simulink model "ErskineMultiDroneFormation"  (R2020b)
settings: Solver=FixedStepAuto  StartTime=0.0  StopTime=Tsim  FixedStep=sim_dt  RelTol=1e-3
values from neighbouring files (symbols this model uses):
  controller_rate = 50    [MultiQuadInit.m]
  drone_params = setDefaultDroneParams(nDrones)    [MultiQuadInit.m]
  dt_p = 0.2    [MultiQuadInit.m]    (also in setSimConditions.m)
  edges = [1,2 ... (first row only)    [MultiQuadInit.m]    (also in setSimConditions.m)
  g = 9.81    [MultiQuadInit.m]
  N_p = 5    [MultiQuadInit.m]    (also in setSimConditions.m)
  nDrones = 3    [MultiQuadInit.m]
  omega0 = zeros(3,nDrones)    [MultiQuadInit.m]    (also in setSimConditions.m)
  p0 = scale*(rand(3,nDrones) - [0.5;0.5;0])    [MultiQuadInit.m]    (also in setSimConditions.m = scale*(rand(3,nDrones) - [1/2;1/2;0]))
  q0 = zeros(4,nDrones); q0(1,:) = ones(1,nDrones)    [MultiQuadInit.m]    (also in setSimConditions.m)
  sim_dt = 0.005    [MultiQuadInit.m]
  v0 = zeros(3, nDrones)    [MultiQuadInit.m]    (also in setSimConditions.m)
undefined symbols (not defined in the file or in its folder): camera_noise
libraries: vrlib x13
(part 2 of 4)

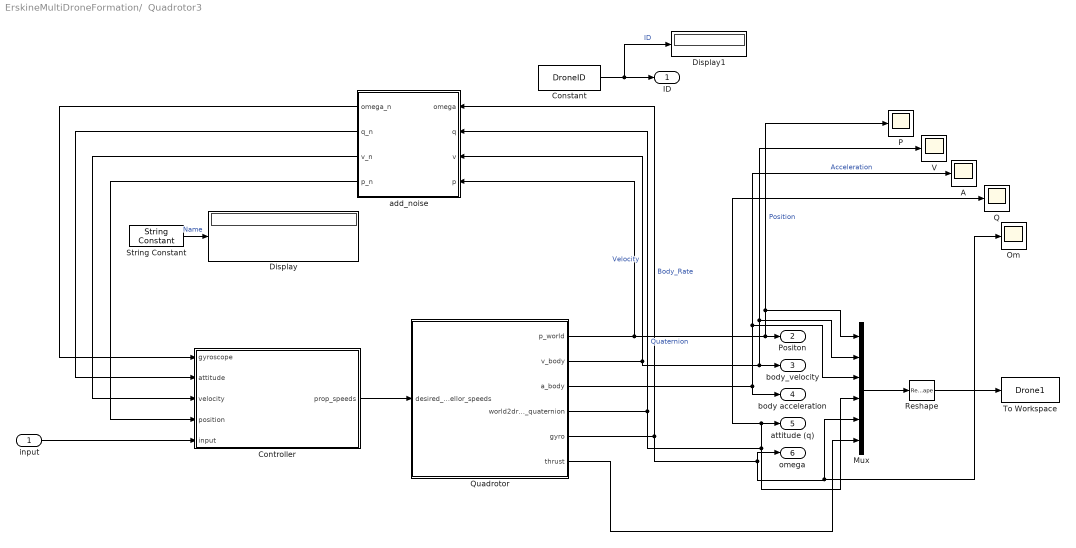
== system ErskineMultiDroneFormation/  Quadrotor3 ==
  input : Inport
  A : Scope
  Constant : Constant  Value=DroneID
  Controller : Subsystem
      mask Display: image('Format/flightController.png'); % Use "Edit Image" on toolstrip to change.
  Display : Display
  Display1 : Display
  Mux : Mux  Inputs=6
  Om : Scope
  P : Scope
  Q : Scope
  Quadrotor : Subsystem
      mask Display: image('droneHardware.jpeg'); % Use "Edit Image" on toolstrip to change.
  Reshape : Reshape
  String Constant : StringConstant  String=DroneName
  To Workspace : ToWorkspace  VariableName=Drone1  SaveFormat=Timeseries  SampleTime=-1
  V : Scope
  add_noise : MATLAB Function  TreatAsAtomicUnit=on
  ID : Outport
  Positon : Outport  Port=2
  body_velocity : Outport  Port=3
  body acceleration : Outport  Port=4
  attitude (q) : Outport  Port=5
  omega : Outport  Port=6
  wires:
  Quadrotor/5(gyro) -> Om/1, Mux/5, omega/1, add_noise/1(omega)  "Body_Rate"
  Quadrotor/1(p_world) -> add_noise/4(p), P/1, Mux/1, Positon/1  "Position"
  Quadrotor/3(a_body) -> body acceleration/1, A/1, Mux/3  "Acceleration"
  Quadrotor/4(world2drone_quaternion) -> Q/1, attitude (q)/1, Mux/4, add_noise/2(q)  "Quaternion"
  Mux/1 -> Reshape/1
  Quadrotor/2(v_body) -> V/1, Mux/2, body_velocity/1, add_noise/3(v)  "Velocity"
  Quadrotor/6(thrust) -> Mux/6
  String Constant/1 -> Display/1  "Name"
  Constant/1 -> Display1/1, ID/1  "ID"
  Reshape/1 -> To Workspace/1
  add_noise/1(omega_n) -> Controller/1(gyroscope)
  add_noise/2(q_n) -> Controller/2(attitude)
  add_noise/3(v_n) -> Controller/3(velocity)
  add_noise/4(p_n) -> Controller/4(position)
  input/1 -> Controller/5(input)
  Controller/1(prop_speeds) -> Quadrotor/1(desired_propellor_speeds)

== system ErskineMultiDroneFormation/  Quadrotor4 ==
  input : Inport
  A : Scope
  Constant : Constant  Value=DroneID
  Controller : Subsystem
      mask Display: image('Format/flightController.png'); % Use "Edit Image" on toolstrip to change.
  Display : Display
  Display1 : Display
  Mux : Mux  Inputs=6
  Om : Scope
  P : Scope
  Q : Scope
  Quadrotor : Subsystem
      mask Display: image('droneHardware.jpeg'); % Use "Edit Image" on toolstrip to change.
  Reshape : Reshape
  String Constant : StringConstant  String=DroneName
  To Workspace : ToWorkspace  VariableName=Drone5  SaveFormat=Timeseries  SampleTime=-1
  V : Scope
  add_noise : MATLAB Function  TreatAsAtomicUnit=on
  ID : Outport
  Positon : Outport  Port=2
  body_velocity : Outport  Port=3
  body acceleration : Outport  Port=4
  attitude (q) : Outport  Port=5
  omega : Outport  Port=6
  wires:
  Quadrotor/5(gyro) -> Om/1, Mux/5, omega/1, add_noise/1(omega)  "Body_Rate"
  Quadrotor/1(p_world) -> add_noise/4(p), P/1, Mux/1, Positon/1  "Position"
  Quadrotor/3(a_body) -> body acceleration/1, A/1, Mux/3  "Acceleration"
  Quadrotor/4(world2drone_quaternion) -> Q/1, attitude (q)/1, Mux/4, add_noise/2(q)  "Quaternion"
  Mux/1 -> Reshape/1
  Quadrotor/2(v_body) -> V/1, Mux/2, body_velocity/1, add_noise/3(v)  "Velocity"
  Quadrotor/6(thrust) -> Mux/6
  String Constant/1 -> Display/1  "Name"
  Constant/1 -> Display1/1, ID/1  "ID"
  Reshape/1 -> To Workspace/1
  add_noise/1(omega_n) -> Controller/1(gyroscope)
  add_noise/2(q_n) -> Controller/2(attitude)
  add_noise/3(v_n) -> Controller/3(velocity)
  add_noise/4(p_n) -> Controller/4(position)
  input/1 -> Controller/5(input)
  Controller/1(prop_speeds) -> Quadrotor/1(desired_propellor_speeds)

== system ErskineMultiDroneFormation/  Quadrotor5 ==
  input : Inport
  A : Scope
  Constant : Constant  Value=DroneID
  Controller : Subsystem
      mask Display: image('Format/flightController.png'); % Use "Edit Image" on toolstrip to change.
  Display : Display
  Display1 : Display
  Mux : Mux  Inputs=6
  Om : Scope
  P : Scope
  Q : Scope
  Quadrotor : Subsystem
      mask Display: image('droneHardware.jpeg'); % Use "Edit Image" on toolstrip to change.
  Reshape : Reshape
  String Constant : StringConstant  String=DroneName
  To Workspace : ToWorkspace  VariableName=Drone6  SaveFormat=Timeseries  SampleTime=-1
  V : Scope
  add_noise : MATLAB Function  TreatAsAtomicUnit=on
  ID : Outport
  Positon : Outport  Port=2
  body_velocity : Outport  Port=3
  body acceleration : Outport  Port=4
  attitude (q) : Outport  Port=5
  omega : Outport  Port=6
  wires:
  Quadrotor/5(gyro) -> Om/1, Mux/5, omega/1, add_noise/1(omega)  "Body_Rate"
  Quadrotor/1(p_world) -> add_noise/4(p), P/1, Mux/1, Positon/1  "Position"
  Quadrotor/3(a_body) -> body acceleration/1, A/1, Mux/3  "Acceleration"
  Quadrotor/4(world2drone_quaternion) -> Q/1, attitude (q)/1, Mux/4, add_noise/2(q)  "Quaternion"
  Mux/1 -> Reshape/1
  Quadrotor/2(v_body) -> V/1, Mux/2, body_velocity/1, add_noise/3(v)  "Velocity"
  Quadrotor/6(thrust) -> Mux/6
  String Constant/1 -> Display/1  "Name"
  Constant/1 -> Display1/1, ID/1  "ID"
  Reshape/1 -> To Workspace/1
  add_noise/1(omega_n) -> Controller/1(gyroscope)
  add_noise/2(q_n) -> Controller/2(attitude)
  add_noise/3(v_n) -> Controller/3(velocity)
  add_noise/4(p_n) -> Controller/4(position)
  input/1 -> Controller/5(input)
  Controller/1(prop_speeds) -> Quadrotor/1(desired_propellor_speeds)

== system ErskineMultiDroneFormation/  Quadrotor6 ==
  input : Inport
  A : Scope
  Constant : Constant  Value=DroneID
  Controller : Subsystem
      mask Display: image('Format/flightController.png'); % Use "Edit Image" on toolstrip to change.
  Display : Display
  Display1 : Display
  Mux : Mux  Inputs=6
  Om : Scope
  P : Scope
  Q : Scope
  Quadrotor : Subsystem
      mask Display: image('droneHardware.jpeg'); % Use "Edit Image" on toolstrip to change.
  Reshape : Reshape
  String Constant : StringConstant  String=DroneName
  To Workspace : ToWorkspace  VariableName=Drone4  SaveFormat=Timeseries  SampleTime=-1
  V : Scope
  add_noise : MATLAB Function  TreatAsAtomicUnit=on
  ID : Outport
  Positon : Outport  Port=2
  body_velocity : Outport  Port=3
  body acceleration : Outport  Port=4
  attitude (q) : Outport  Port=5
  omega : Outport  Port=6
  wires:
  Quadrotor/5(gyro) -> Om/1, Mux/5, omega/1, add_noise/1(omega)  "Body_Rate"
  Quadrotor/1(p_world) -> add_noise/4(p), P/1, Mux/1, Positon/1  "Position"
  Quadrotor/3(a_body) -> body acceleration/1, A/1, Mux/3  "Acceleration"
  Quadrotor/4(world2drone_quaternion) -> Q/1, attitude (q)/1, Mux/4, add_noise/2(q)  "Quaternion"
  Mux/1 -> Reshape/1
  Quadrotor/2(v_body) -> V/1, Mux/2, body_velocity/1, add_noise/3(v)  "Velocity"
  Quadrotor/6(thrust) -> Mux/6
  String Constant/1 -> Display/1  "Name"
  Constant/1 -> Display1/1, ID/1  "ID"
  Reshape/1 -> To Workspace/1
  add_noise/1(omega_n) -> Controller/1(gyroscope)
  add_noise/2(q_n) -> Controller/2(attitude)
  add_noise/3(v_n) -> Controller/3(velocity)
  add_noise/4(p_n) -> Controller/4(position)
  input/1 -> Controller/5(input)
  Controller/1(prop_speeds) -> Quadrotor/1(desired_propellor_speeds)

== system ErskineMultiDroneFormation/  Quadrotor7 ==
  input : Inport
  A : Scope
  Constant : Constant  Value=DroneID
  Controller : Subsystem
      mask Display: image('Format/flightController.png'); % Use "Edit Image" on toolstrip to change.
  Display : Display
  Display1 : Display
  Mux : Mux  Inputs=6
  Om : Scope
  P : Scope
  Q : Scope
  Quadrotor : Subsystem
      mask Display: image('droneHardware.jpeg'); % Use "Edit Image" on toolstrip to change.
  Reshape : Reshape
  String Constant : StringConstant  String=DroneName
  To Workspace : ToWorkspace  VariableName=Drone8  SaveFormat=Timeseries  SampleTime=-1
  V : Scope
  add_noise : MATLAB Function  TreatAsAtomicUnit=on
  ID : Outport
  Positon : Outport  Port=2
  body_velocity : Outport  Port=3
  body acceleration : Outport  Port=4
  attitude (q) : Outport  Port=5
  omega : Outport  Port=6
  wires:
  Quadrotor/5(gyro) -> Om/1, Mux/5, omega/1, add_noise/1(omega)  "Body_Rate"
  Quadrotor/1(p_world) -> add_noise/4(p), P/1, Mux/1, Positon/1  "Position"
  Quadrotor/3(a_body) -> body acceleration/1, A/1, Mux/3  "Acceleration"
  Quadrotor/4(world2drone_quaternion) -> Q/1, attitude (q)/1, Mux/4, add_noise/2(q)  "Quaternion"
  Mux/1 -> Reshape/1
  Quadrotor/2(v_body) -> V/1, Mux/2, body_velocity/1, add_noise/3(v)  "Velocity"
  Quadrotor/6(thrust) -> Mux/6
  String Constant/1 -> Display/1  "Name"
  Constant/1 -> Display1/1, ID/1  "ID"
  Reshape/1 -> To Workspace/1
  add_noise/1(omega_n) -> Controller/1(gyroscope)
  add_noise/2(q_n) -> Controller/2(attitude)
  add_noise/3(v_n) -> Controller/3(velocity)
  add_noise/4(p_n) -> Controller/4(position)
  input/1 -> Controller/5(input)
  Controller/1(prop_speeds) -> Quadrotor/1(desired_propellor_speeds)

== system ErskineMultiDroneFormation/  Quadrotor8 ==
  input : Inport
  A : Scope
  Constant : Constant  Value=DroneID
  Controller : Subsystem
      mask Display: image('Format/flightController.png'); % Use "Edit Image" on toolstrip to change.
  Display : Display
  Display1 : Display
  Mux : Mux  Inputs=6
  Om : Scope
  P : Scope
  Q : Scope
  Quadrotor : Subsystem
      mask Display: image('droneHardware.jpeg'); % Use "Edit Image" on toolstrip to change.
  Reshape : Reshape
  String Constant : StringConstant  String=DroneName
  To Workspace : ToWorkspace  VariableName=Drone9  SaveFormat=Timeseries  SampleTime=-1
  V : Scope
  add_noise : MATLAB Function  TreatAsAtomicUnit=on
  ID : Outport
  Positon : Outport  Port=2
  body_velocity : Outport  Port=3
  body acceleration : Outport  Port=4
  attitude (q) : Outport  Port=5
  omega : Outport  Port=6
  wires:
  Quadrotor/5(gyro) -> Om/1, Mux/5, omega/1, add_noise/1(omega)  "Body_Rate"
  Quadrotor/1(p_world) -> add_noise/4(p), P/1, Mux/1, Positon/1  "Position"
  Quadrotor/3(a_body) -> body acceleration/1, A/1, Mux/3  "Acceleration"
  Quadrotor/4(world2drone_quaternion) -> Q/1, attitude (q)/1, Mux/4, add_noise/2(q)  "Quaternion"
  Mux/1 -> Reshape/1
  Quadrotor/2(v_body) -> V/1, Mux/2, body_velocity/1, add_noise/3(v)  "Velocity"
  Quadrotor/6(thrust) -> Mux/6
  String Constant/1 -> Display/1  "Name"
  Constant/1 -> Display1/1, ID/1  "ID"
  Reshape/1 -> To Workspace/1
  add_noise/1(omega_n) -> Controller/1(gyroscope)
  add_noise/2(q_n) -> Controller/2(attitude)
  add_noise/3(v_n) -> Controller/3(velocity)
  add_noise/4(p_n) -> Controller/4(position)
  input/1 -> Controller/5(input)
  Controller/1(prop_speeds) -> Quadrotor/1(desired_propellor_speeds)

== system ErskineMultiDroneFormation/  Quadrotor9 ==
  input : Inport
  A : Scope
  Constant : Constant  Value=DroneID
  Controller : Subsystem
      mask Display: image('Format/flightController.png'); % Use "Edit Image" on toolstrip to change.
  Display : Display
  Display1 : Display
  Mux : Mux  Inputs=6
  Om : Scope
  P : Scope
  Q : Scope
  Quadrotor : Subsystem
      mask Display: image('droneHardware.jpeg'); % Use "Edit Image" on toolstrip to change.
  Reshape : Reshape
  String Constant : StringConstant  String=DroneName
  To Workspace : ToWorkspace  VariableName=Drone7  SaveFormat=Timeseries  SampleTime=-1
  V : Scope
  add_noise : MATLAB Function  TreatAsAtomicUnit=on
  ID : Outport
  Positon : Outport  Port=2
  body_velocity : Outport  Port=3
  body acceleration : Outport  Port=4
  attitude (q) : Outport  Port=5
  omega : Outport  Port=6
  wires:
  Quadrotor/5(gyro) -> Om/1, Mux/5, omega/1, add_noise/1(omega)  "Body_Rate"
  Quadrotor/1(p_world) -> add_noise/4(p), P/1, Mux/1, Positon/1  "Position"
  Quadrotor/3(a_body) -> body acceleration/1, A/1, Mux/3  "Acceleration"
  Quadrotor/4(world2drone_quaternion) -> Q/1, attitude (q)/1, Mux/4, add_noise/2(q)  "Quaternion"
  Mux/1 -> Reshape/1
  Quadrotor/2(v_body) -> V/1, Mux/2, body_velocity/1, add_noise/3(v)  "Velocity"
  Quadrotor/6(thrust) -> Mux/6
  String Constant/1 -> Display/1  "Name"
  Constant/1 -> Display1/1, ID/1  "ID"
  Reshape/1 -> To Workspace/1
  add_noise/1(omega_n) -> Controller/1(gyroscope)
  add_noise/2(q_n) -> Controller/2(attitude)
  add_noise/3(v_n) -> Controller/3(velocity)
  add_noise/4(p_n) -> Controller/4(position)
  input/1 -> Controller/5(input)
  Controller/1(prop_speeds) -> Quadrotor/1(desired_propellor_speeds)

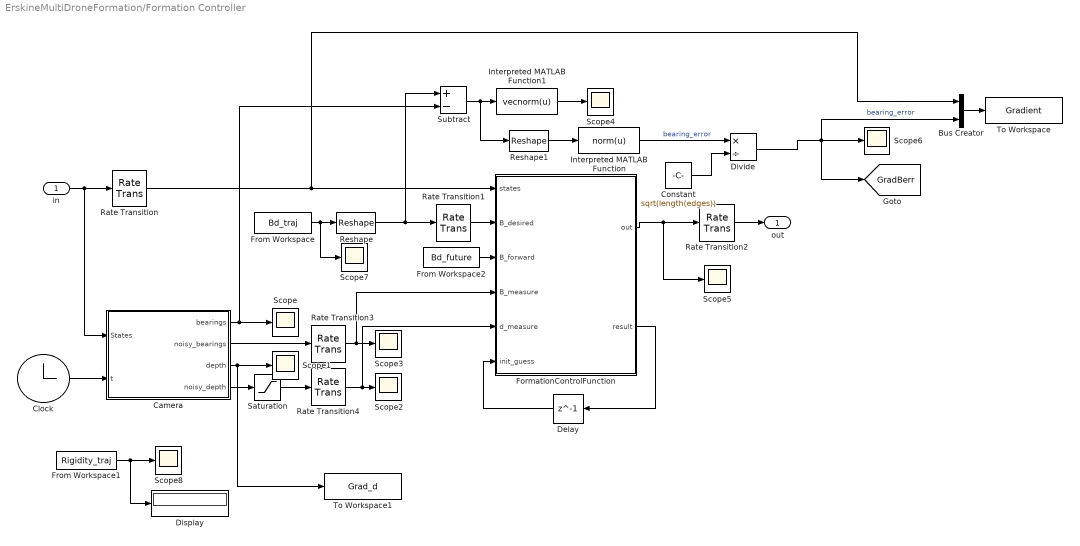
== system ErskineMultiDroneFormation/Formation Controller ==
  in : Inport
  Bus Creator : BusCreator  Inputs=2
  Camera : MATLAB Function  TreatAsAtomicUnit=on  SystemSampleTime=sim_dt
  Clock : Clock
  Constant : Constant  Value=sqrt(length(edges))
  Delay : Delay  DelayLength=1  InitialCondition=zeros(nDrones*4*N_p, 1)
  Display : Display
  Divide : Product  Inputs=*/
  FormationControlFunction : MATLAB Function  TreatAsAtomicUnit=on
  From Workspace : FromWorkspace  VariableName=Bd_traj  SampleTime=sim_dt  OutputAfterFinalValue=Holding final value
  From Workspace1 : FromWorkspace  VariableName=Rigidity_traj  SampleTime=sim_dt  OutputAfterFinalValue=Holding final value
  From Workspace2 : FromWorkspace  VariableName=Bd_future  SampleTime=sim_dt  OutputAfterFinalValue=Holding final value
  Interpreted MATLAB Function : MATLABFcn  MATLABFcn=norm(u)
  Interpreted MATLAB Function1 : MATLABFcn  MATLABFcn=vecnorm(u)
  Rate Transition{,1,3..4} (4 alike) : RateTransition  OutPortSampleTime=1/controller_rate
  Rate Transition2 : RateTransition  OutPortSampleTime=sim_dt
  Reshape : Reshape  OutputDimensionality=Customize  OutputDimensions=[3,length(edges)]
  Reshape1 : Reshape  OutputDimensions=[3,length(edges)]
  Saturation : Saturate  UpperLimit=999999  LowerLimit=0.2
  Scope{,1..8} (9 alike) : Scope
  Subtract : Sum  Inputs=+-
  To Workspace : ToWorkspace  VariableName=Gradient  SaveFormat=Timeseries  SampleTime=-1
  To Workspace1 : ToWorkspace  VariableName=Grad_d  SaveFormat=Timeseries  SampleTime=-1
  out : Outport
  tag scope: GradBerr=global
  wires:
  in/1 -> Camera/1(States), Rate Transition/1
  FormationControlFunction/1(out) -> Scope5/1, Rate Transition2/1
  FormationControlFunction/2(result) -> Delay/1
  Delay/1 -> FormationControlFunction/6(init_guess)
  Camera/1(bearings) -> Scope/1, Subtract/2
  Rate Transition/1 -> Bus Creator/1, FormationControlFunction/1(states)
  Rate Transition1/1 -> FormationControlFunction/2(B_desired)
  Rate Transition2/1 -> out/1
  Camera/3(depth) -> To Workspace1/1, Scope1/1
  Camera/4(noisy_depth) -> Saturation/1
  Camera/2(noisy_bearings) -> Rate Transition3/1
  Rate Transition3/1 -> FormationControlFunction/4(B_measure), Scope3/1
  Rate Transition4/1 -> FormationControlFunction/5(d_measure), Scope2/1
  Reshape/1 -> Rate Transition1/1, Subtract/1
  Subtract/1 -> Reshape1/1, Interpreted MATLAB Function1/1
  Reshape1/1 -> Interpreted MATLAB Function/1
  Saturation/1 -> Rate Transition4/1
  From Workspace/1 -> Scope7/1, Reshape/1
  Clock/1 -> Camera/2(t)
  Interpreted MATLAB Function1/1 -> Scope4/1
  From Workspace1/1 -> Display/1, Scope8/1
  From Workspace2/1 -> FormationControlFunction/3(B_forward)
  Bus Creator/1 -> To Workspace/1
  Divide/1 -> [GradBerr], Bus Creator/2, Scope6/1  "bearing_error"
  Constant/1 -> Divide/2
  Interpreted MATLAB Function/1 -> Divide/1  "bearing_error"

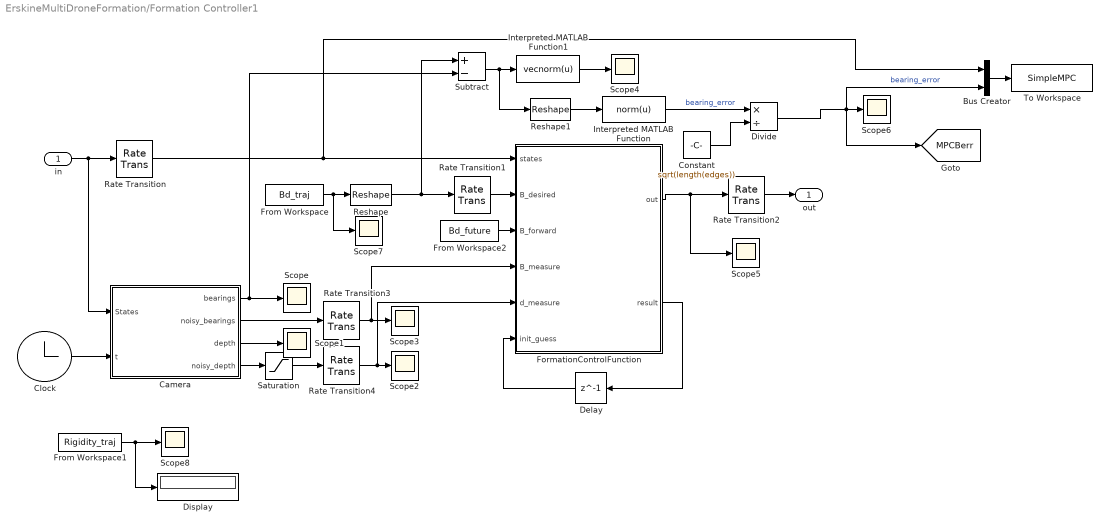
== system ErskineMultiDroneFormation/Formation Controller1 ==
  in : Inport
  Bus Creator : BusCreator  Inputs=2
  Camera : MATLAB Function  TreatAsAtomicUnit=on  SystemSampleTime=sim_dt
  Clock : Clock
  Constant : Constant  Value=sqrt(length(edges))
  Delay : Delay  DelayLength=1  InitialCondition=zeros(nDrones*4*N_p, 1)
  Display : Display
  Divide : Product  Inputs=*/
  FormationControlFunction : MATLAB Function  TreatAsAtomicUnit=on
  From Workspace : FromWorkspace  VariableName=Bd_traj  SampleTime=sim_dt  OutputAfterFinalValue=Holding final value
  From Workspace1 : FromWorkspace  VariableName=Rigidity_traj  SampleTime=sim_dt  OutputAfterFinalValue=Holding final value
  From Workspace2 : FromWorkspace  VariableName=Bd_future  SampleTime=sim_dt  OutputAfterFinalValue=Holding final value
  Interpreted MATLAB Function : MATLABFcn  MATLABFcn=norm(u)
  Interpreted MATLAB Function1 : MATLABFcn  MATLABFcn=vecnorm(u)
  Rate Transition{,1,3..4} (4 alike) : RateTransition  OutPortSampleTime=1/controller_rate
  Rate Transition2 : RateTransition  OutPortSampleTime=sim_dt
  Reshape : Reshape  OutputDimensionality=Customize  OutputDimensions=[3,length(edges)]
  Reshape1 : Reshape  OutputDimensions=[3,length(edges)]
  Saturation : Saturate  UpperLimit=999999  LowerLimit=0.2
  Scope{,1..8} (9 alike) : Scope
  Subtract : Sum  Inputs=+-
  To Workspace : ToWorkspace  VariableName=SimpleMPC  SaveFormat=Timeseries  SampleTime=-1
  out : Outport
  tag scope: MPCBerr=global
  wires:
  in/1 -> Camera/1(States), Rate Transition/1
  FormationControlFunction/1(out) -> Scope5/1, Rate Transition2/1
  FormationControlFunction/2(result) -> Delay/1
  Delay/1 -> FormationControlFunction/6(init_guess)
  Camera/1(bearings) -> Scope/1, Subtract/2
  Rate Transition/1 -> Bus Creator/1, FormationControlFunction/1(states)
  Rate Transition1/1 -> FormationControlFunction/2(B_desired)
  Rate Transition2/1 -> out/1
  Camera/3(depth) -> Scope1/1
  Camera/4(noisy_depth) -> Saturation/1
  Camera/2(noisy_bearings) -> Rate Transition3/1
  Rate Transition3/1 -> FormationControlFunction/4(B_measure), Scope3/1
  Rate Transition4/1 -> FormationControlFunction/5(d_measure), Scope2/1
  Reshape/1 -> Rate Transition1/1, Subtract/1
  Subtract/1 -> Reshape1/1, Interpreted MATLAB Function1/1
  Reshape1/1 -> Interpreted MATLAB Function/1
  Saturation/1 -> Rate Transition4/1
  From Workspace/1 -> Scope7/1, Reshape/1
  Clock/1 -> Camera/2(t)
  Interpreted MATLAB Function1/1 -> Scope4/1
  From Workspace1/1 -> Display/1, Scope8/1
  From Workspace2/1 -> FormationControlFunction/3(B_forward)
  Bus Creator/1 -> To Workspace/1
  Interpreted MATLAB Function/1 -> Divide/1  "bearing_error"
  Constant/1 -> Divide/2
  Divide/1 -> [MPCBerr], Bus Creator/2, Scope6/1  "bearing_error"

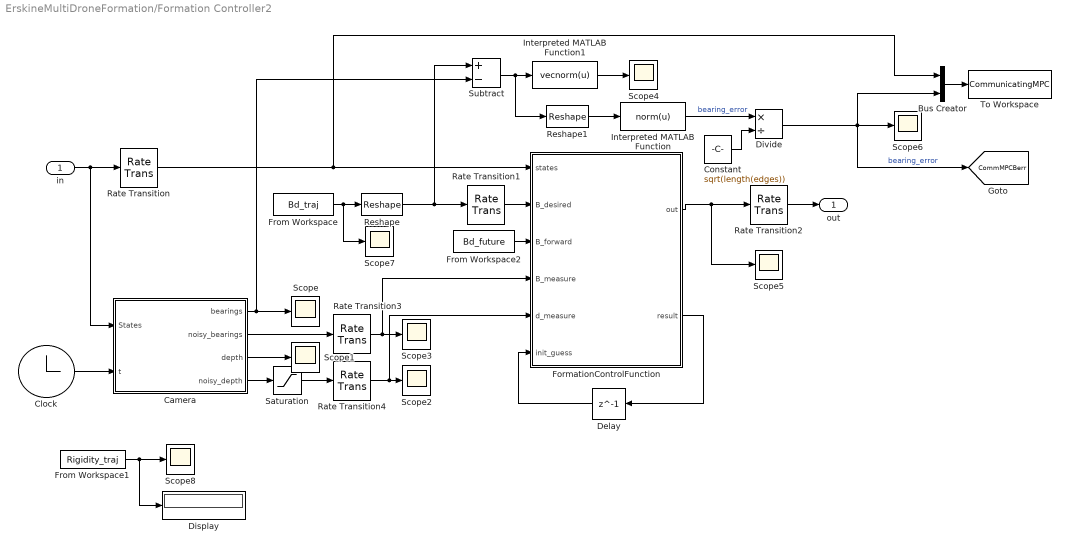
== system ErskineMultiDroneFormation/Formation Controller2 ==
  in : Inport
  Bus Creator : BusCreator  Inputs=2
  Camera : MATLAB Function  TreatAsAtomicUnit=on  SystemSampleTime=sim_dt
  Clock : Clock
  Constant : Constant  Value=sqrt(length(edges))
  Delay : Delay  DelayLength=1  InitialCondition=zeros(nDrones*4*N_p, 1)
  Display : Display
  Divide : Product  Inputs=*/
  FormationControlFunction : MATLAB Function  TreatAsAtomicUnit=on
  From Workspace : FromWorkspace  VariableName=Bd_traj  SampleTime=sim_dt  OutputAfterFinalValue=Holding final value
  From Workspace1 : FromWorkspace  VariableName=Rigidity_traj  SampleTime=sim_dt  OutputAfterFinalValue=Holding final value
  From Workspace2 : FromWorkspace  VariableName=Bd_future  SampleTime=sim_dt  OutputAfterFinalValue=Holding final value
  Interpreted MATLAB Function : MATLABFcn  MATLABFcn=norm(u)
  Interpreted MATLAB Function1 : MATLABFcn  MATLABFcn=vecnorm(u)
  Rate Transition{,1,3..4} (4 alike) : RateTransition  OutPortSampleTime=1/controller_rate
  Rate Transition2 : RateTransition  OutPortSampleTime=sim_dt
  Reshape : Reshape  OutputDimensionality=Customize  OutputDimensions=[3,length(edges)]
  Reshape1 : Reshape  OutputDimensions=[3,length(edges)]
  Saturation : Saturate  UpperLimit=999999  LowerLimit=0.2
  Scope{,1..8} (9 alike) : Scope
  Subtract : Sum  Inputs=+-
  To Workspace : ToWorkspace  VariableName=CommunicatingMPC  SaveFormat=Timeseries  SampleTime=-1
  out : Outport
  tag scope: CommMPCBerr=global
  wires:
  in/1 -> Camera/1(States), Rate Transition/1
  FormationControlFunction/1(out) -> Scope5/1, Rate Transition2/1
  FormationControlFunction/2(result) -> Delay/1
  Delay/1 -> FormationControlFunction/6(init_guess)
  Camera/1(bearings) -> Scope/1, Subtract/2
  Rate Transition/1 -> Bus Creator/1, FormationControlFunction/1(states)
  Rate Transition1/1 -> FormationControlFunction/2(B_desired)
  Rate Transition2/1 -> out/1
  Camera/3(depth) -> Scope1/1
  Camera/4(noisy_depth) -> Saturation/1
  Camera/2(noisy_bearings) -> Rate Transition3/1
  Rate Transition3/1 -> FormationControlFunction/4(B_measure), Scope3/1
  Rate Transition4/1 -> FormationControlFunction/5(d_measure), Scope2/1
  Reshape/1 -> Rate Transition1/1, Subtract/1
  Subtract/1 -> Reshape1/1, Interpreted MATLAB Function1/1
  Reshape1/1 -> Interpreted MATLAB Function/1
  Saturation/1 -> Rate Transition4/1
  From Workspace/1 -> Scope7/1, Reshape/1
  Clock/1 -> Camera/2(t)
  Interpreted MATLAB Function1/1 -> Scope4/1
  From Workspace1/1 -> Display/1, Scope8/1
  From Workspace2/1 -> FormationControlFunction/3(B_forward)
  Bus Creator/1 -> To Workspace/1
  Divide/1 -> [CommMPCBerr], Bus Creator/2, Scope6/1  "bearing_error"
  Constant/1 -> Divide/2
  Interpreted MATLAB Function/1 -> Divide/1  "bearing_error"

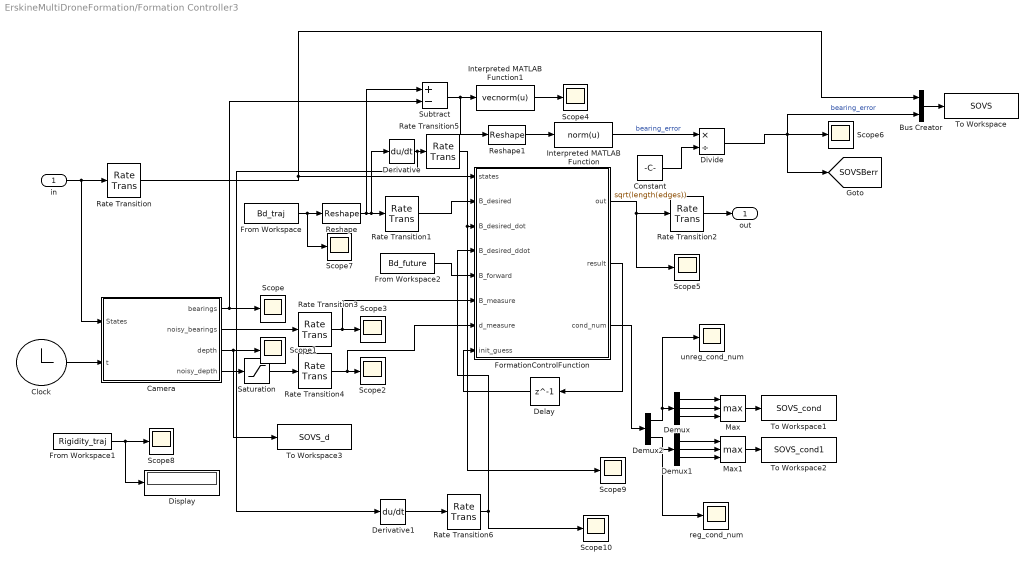
== system ErskineMultiDroneFormation/Formation Controller3 ==
  in : Inport
  Bus Creator : BusCreator  Inputs=2
  Camera : MATLAB Function  TreatAsAtomicUnit=on  SystemSampleTime=sim_dt
  Clock : Clock
  Constant : Constant  Value=sqrt(length(edges))
  Delay : Delay  DelayLength=1  InitialCondition=zeros(nDrones*4*N_p, 1)
  Demux : Demux  Outputs=3
  Demux1 : Demux  Outputs=3
  Demux2 : Demux  Outputs=2
  Derivative : Derivative
  Derivative1 : Derivative
  Display : Display
  Divide : Product  Inputs=*/
  FormationControlFunction : MATLAB Function  TreatAsAtomicUnit=on
  From Workspace : FromWorkspace  VariableName=Bd_traj  SampleTime=sim_dt  OutputAfterFinalValue=Holding final value
  From Workspace1 : FromWorkspace  VariableName=Rigidity_traj  SampleTime=sim_dt  OutputAfterFinalValue=Holding final value
  From Workspace2 : FromWorkspace  VariableName=Bd_future  SampleTime=sim_dt  OutputAfterFinalValue=Holding final value
  Interpreted MATLAB Function : MATLABFcn  MATLABFcn=norm(u)
  Interpreted MATLAB Function1 : MATLABFcn  MATLABFcn=vecnorm(u)
  Max : MinMax  Function=max  Inputs=3
  Max1 : MinMax  Function=max  Inputs=3
  Rate Transition{,1,3..6} (6 alike) : RateTransition  OutPortSampleTime=1/controller_rate
  Rate Transition2 : RateTransition  OutPortSampleTime=sim_dt
  Reshape : Reshape  OutputDimensionality=Customize  OutputDimensions=[3,length(edges)]
  Reshape1 : Reshape  OutputDimensions=[3,length(edges)]
  Saturation : Saturate  UpperLimit=999999  LowerLimit=0.2
  Scope{,1..10} (11 alike) : Scope
  Subtract : Sum  Inputs=+-
  To Workspace : ToWorkspace  VariableName=SOVS  SaveFormat=Timeseries  SampleTime=-1
  To Workspace1 : ToWorkspace  VariableName=SOVS_cond  SaveFormat=Timeseries  SampleTime=-1
  To Workspace2 : ToWorkspace  VariableName=SOVS_cond1  SaveFormat=Timeseries  SampleTime=-1
  To Workspace3 : ToWorkspace  VariableName=SOVS_d  SaveFormat=Timeseries  SampleTime=-1
  reg_cond_num : Scope
  unreg_cond_num : Scope
  out : Outport
  tag scope: SOVSBerr=global
  wires:
  in/1 -> Camera/1(States), Rate Transition/1
  FormationControlFunction/1(out) -> Scope5/1, Rate Transition2/1
  FormationControlFunction/2(result) -> Delay/1
  Delay/1 -> FormationControlFunction/8(init_guess)
  Camera/1(bearings) -> Scope/1, Subtract/2
  Rate Transition/1 -> Bus Creator/1, FormationControlFunction/1(states)
  Rate Transition1/1 -> FormationControlFunction/2(B_desired)
  Rate Transition2/1 -> out/1
  Camera/3(depth) -> To Workspace3/1, Scope1/1
  Camera/4(noisy_depth) -> Saturation/1
  Camera/2(noisy_bearings) -> Rate Transition3/1
  Rate Transition3/1 -> FormationControlFunction/6(B_measure), Scope3/1
  Rate Transition4/1 -> FormationControlFunction/7(d_measure), Scope2/1
  Reshape/1 -> Derivative/1, Rate Transition1/1, Subtract/1
  Subtract/1 -> Reshape1/1, Interpreted MATLAB Function1/1
  Reshape1/1 -> Interpreted MATLAB Function/1
  Saturation/1 -> Rate Transition4/1
  From Workspace/1 -> Scope7/1, Reshape/1
  Clock/1 -> Camera/2(t)
  Interpreted MATLAB Function1/1 -> Scope4/1
  From Workspace1/1 -> Display/1, Scope8/1
  From Workspace2/1 -> FormationControlFunction/5(B_forward)
  Bus Creator/1 -> To Workspace/1
  Divide/1 -> [SOVSBerr], Bus Creator/2, Scope6/1  "bearing_error"
  Constant/1 -> Divide/2
  Interpreted MATLAB Function/1 -> Divide/1  "bearing_error"
  Derivative/1 -> Derivative1/1, Rate Transition5/1
  Rate Transition5/1 -> Scope9/1, FormationControlFunction/3(B_desired_dot)
  Derivative1/1 -> Rate Transition6/1
  Rate Transition6/1 -> Scope10/1, FormationControlFunction/4(B_desired_ddot)
  FormationControlFunction/3(cond_num) -> Demux2/1
  Demux/1 -> Max/1
  Demux/2 -> Max/2
  Demux/3 -> Max/3
  Max/1 -> To Workspace1/1
  Demux1/2 -> Max1/2
  Demux1/1 -> Max1/1
  Demux1/3 -> Max1/3
  Max1/1 -> To Workspace2/1
  Demux2/1 -> unreg_cond_num/1, Demux/1
  Demux2/2 -> reg_cond_num/1, Demux1/1

== system ErskineMultiDroneFormation/  Quadrotor1/Controller ==
  gyroscope : Inport
  attitude : Inport  Port=2
  velocity : Inport  Port=3
  position : Inport  Port=4
  input : Inport  Port=5
  Controller : MATLAB Function  TreatAsAtomicUnit=on
  Saturation : Saturate  UpperLimit=drone_params(DroneID).control.limits.thrust.max  LowerLimit=drone_params(DroneID).control.limits.thrust.min
  Saturation1 : Saturate  UpperLimit=0.1  LowerLimit=-0.1
  desired_prop_speed : MATLAB Function  TreatAsAtomicUnit=on
  prop_speeds : Outport
  wires:
  Controller/2(moments) -> Saturation1/1
  Saturation/1 -> desired_prop_speed/1(thrust)
  velocity/1 -> Controller/3(v)
  Saturation1/1 -> desired_prop_speed/2(moment)
  Controller/1(thrust) -> Saturation/1
  position/1 -> Controller/2(p)
  input/1 -> Controller/1(u)
  attitude/1 -> Controller/4(q)
  gyroscope/1 -> Controller/5(omega)
  desired_prop_speed/1(Omega_props) -> prop_speeds/1

== system ErskineMultiDroneFormation/  Quadrotor1/Quadrotor ==
  note: Quadrotor_dynamics
  note: Propeller Dynamics
  desired_propellor_speeds : Inport
  Attitude : Subsystem
  ESC : MATLAB Function  TreatAsAtomicUnit=on
  Scope : Scope
  Translation : Subsystem
  calculate_wrench : MATLAB Function  TreatAsAtomicUnit=on
  prop_speed : Integrator  InitialCondition=drone_params(DroneID).motors.omega0  LimitOutput=on  UpperSaturationLimit=drone_params(DroneID).motors.omega_max  LowerSaturationLimit=drone_params(DroneID).motors.omega_min
  prop_speed_scope : Scope
  wrench_scope : Scope  NumInputPorts=2
  p_world : Outport
  v_body : Outport  Port=2
  a_body : Outport  Port=3
  world2drone_quaternion : Outport  Port=4
  gyro : Outport  Port=5
  thrust : Outport  Port=6
  wires:
  calculate_wrench/1(thrust) -> wrench_scope/1, thrust/1, Translation/2(thrust)
  ESC/1(prop_acceleration) -> prop_speed/1
  desired_propellor_speeds/1 -> ESC/1(Omega_prop_d)
  prop_speed/1 -> prop_speed_scope/1, calculate_wrench/1(Omega_props), ESC/2(Omega_prop)
  calculate_wrench/2(moments) -> wrench_scope/2, Attitude/1(body moments)
  Attitude/1(attitude) -> world2drone_quaternion/1, Translation/1(attitude)
  Attitude/2(gyro) -> gyro/1
  Translation/3(body_v) -> v_body/1
  Translation/4(body_a) -> a_body/1
  Translation/1(p) -> p_world/1
  Translation/2(v) -> Scope/1

== system ErskineMultiDroneFormation/  Quadrotor10/Controller ==
  gyroscope : Inport
  attitude : Inport  Port=2
  velocity : Inport  Port=3
  position : Inport  Port=4
  input : Inport  Port=5
  Controller : MATLAB Function  TreatAsAtomicUnit=on
  Saturation : Saturate  UpperLimit=drone_params(DroneID).control.limits.thrust.max  LowerLimit=drone_params(DroneID).control.limits.thrust.min
  Saturation1 : Saturate  UpperLimit=0.1  LowerLimit=-0.1
  desired_prop_speed : MATLAB Function  TreatAsAtomicUnit=on
  prop_speeds : Outport
  wires:
  Controller/2(moments) -> Saturation1/1
  Saturation/1 -> desired_prop_speed/1(thrust)
  velocity/1 -> Controller/3(v)
  Saturation1/1 -> desired_prop_speed/2(moment)
  Controller/1(thrust) -> Saturation/1
  position/1 -> Controller/2(p)
  input/1 -> Controller/1(u)
  attitude/1 -> Controller/4(q)
  gyroscope/1 -> Controller/5(omega)
  desired_prop_speed/1(Omega_props) -> prop_speeds/1

== system ErskineMultiDroneFormation/  Quadrotor10/Quadrotor ==
  note: Quadrotor_dynamics
  note: Propeller Dynamics
  desired_propellor_speeds : Inport
  Attitude : Subsystem
  ESC : MATLAB Function  TreatAsAtomicUnit=on
  Scope : Scope
  Translation : Subsystem
  calculate_wrench : MATLAB Function  TreatAsAtomicUnit=on
  prop_speed : Integrator  InitialCondition=drone_params(DroneID).motors.omega0  LimitOutput=on  UpperSaturationLimit=drone_params(DroneID).motors.omega_max  LowerSaturationLimit=drone_params(DroneID).motors.omega_min
  prop_speed_scope : Scope
  wrench_scope : Scope  NumInputPorts=2
  p_world : Outport
  v_body : Outport  Port=2
  a_body : Outport  Port=3
  world2drone_quaternion : Outport  Port=4
  gyro : Outport  Port=5
  thrust : Outport  Port=6
  wires:
  calculate_wrench/1(thrust) -> wrench_scope/1, thrust/1, Translation/2(thrust)
  ESC/1(prop_acceleration) -> prop_speed/1
  desired_propellor_speeds/1 -> ESC/1(Omega_prop_d)
  prop_speed/1 -> prop_speed_scope/1, calculate_wrench/1(Omega_props), ESC/2(Omega_prop)
  calculate_wrench/2(moments) -> wrench_scope/2, Attitude/1(body moments)
  Attitude/1(attitude) -> world2drone_quaternion/1, Translation/1(attitude)
  Attitude/2(gyro) -> gyro/1
  Translation/3(body_v) -> v_body/1
  Translation/4(body_a) -> a_body/1
  Translation/1(p) -> p_world/1
  Translation/2(v) -> Scope/1

== system ErskineMultiDroneFormation/  Quadrotor11/Controller ==
  gyroscope : Inport
  attitude : Inport  Port=2
  velocity : Inport  Port=3
  position : Inport  Port=4
  input : Inport  Port=5
  Controller : MATLAB Function  TreatAsAtomicUnit=on
  Saturation : Saturate  UpperLimit=drone_params(DroneID).control.limits.thrust.max  LowerLimit=drone_params(DroneID).control.limits.thrust.min
  Saturation1 : Saturate  UpperLimit=0.1  LowerLimit=-0.1
  desired_prop_speed : MATLAB Function  TreatAsAtomicUnit=on
  prop_speeds : Outport
  wires:
  Controller/2(moments) -> Saturation1/1
  Saturation/1 -> desired_prop_speed/1(thrust)
  velocity/1 -> Controller/3(v)
  Saturation1/1 -> desired_prop_speed/2(moment)
  Controller/1(thrust) -> Saturation/1
  position/1 -> Controller/2(p)
  input/1 -> Controller/1(u)
  attitude/1 -> Controller/4(q)
  gyroscope/1 -> Controller/5(omega)
  desired_prop_speed/1(Omega_props) -> prop_speeds/1

== system ErskineMultiDroneFormation/  Quadrotor11/Quadrotor ==
  note: Quadrotor_dynamics
  note: Propeller Dynamics
  desired_propellor_speeds : Inport
  Attitude : Subsystem
  ESC : MATLAB Function  TreatAsAtomicUnit=on
  Scope : Scope
  Translation : Subsystem
  calculate_wrench : MATLAB Function  TreatAsAtomicUnit=on
  prop_speed : Integrator  InitialCondition=drone_params(DroneID).motors.omega0  LimitOutput=on  UpperSaturationLimit=drone_params(DroneID).motors.omega_max  LowerSaturationLimit=drone_params(DroneID).motors.omega_min
  prop_speed_scope : Scope
  wrench_scope : Scope  NumInputPorts=2
  p_world : Outport
  v_body : Outport  Port=2
  a_body : Outport  Port=3
  world2drone_quaternion : Outport  Port=4
  gyro : Outport  Port=5
  thrust : Outport  Port=6
  wires:
  calculate_wrench/1(thrust) -> wrench_scope/1, thrust/1, Translation/2(thrust)
  ESC/1(prop_acceleration) -> prop_speed/1
  desired_propellor_speeds/1 -> ESC/1(Omega_prop_d)
  prop_speed/1 -> prop_speed_scope/1, calculate_wrench/1(Omega_props), ESC/2(Omega_prop)
  calculate_wrench/2(moments) -> wrench_scope/2, Attitude/1(body moments)
  Attitude/1(attitude) -> world2drone_quaternion/1, Translation/1(attitude)
  Attitude/2(gyro) -> gyro/1
  Translation/3(body_v) -> v_body/1
  Translation/4(body_a) -> a_body/1
  Translation/1(p) -> p_world/1
  Translation/2(v) -> Scope/1

== system ErskineMultiDroneFormation/  Quadrotor12/Controller ==
  gyroscope : Inport
  attitude : Inport  Port=2
  velocity : Inport  Port=3
  position : Inport  Port=4
  input : Inport  Port=5
  Controller : MATLAB Function  TreatAsAtomicUnit=on
  Saturation : Saturate  UpperLimit=16  LowerLimit=3
  Saturation1 : Saturate  UpperLimit=0.1  LowerLimit=-0.1
  desired_prop_speed : MATLAB Function  TreatAsAtomicUnit=on
  prop_speeds : Outport
  wires:
  Controller/2(moments) -> Saturation1/1
  Saturation/1 -> desired_prop_speed/1(thrust)
  velocity/1 -> Controller/3(v)
  Saturation1/1 -> desired_prop_speed/2(moment)
  Controller/1(thrust) -> Saturation/1
  position/1 -> Controller/2(p)
  input/1 -> Controller/1(u)
  attitude/1 -> Controller/4(q)
  gyroscope/1 -> Controller/5(omega)
  desired_prop_speed/1(Omega_props) -> prop_speeds/1

== system ErskineMultiDroneFormation/  Quadrotor12/Quadrotor ==
  note: Quadrotor_dynamics
  note: Propeller Dynamics
  desired_propellor_speeds : Inport
  Attitude : Subsystem
  ESC : MATLAB Function  TreatAsAtomicUnit=on
  Scope : Scope
  Translation : Subsystem
  calculate_wrench : MATLAB Function  TreatAsAtomicUnit=on
  prop_speed : Integrator  InitialCondition=drone_params(DroneID).motors.omega0  LimitOutput=on  UpperSaturationLimit=drone_params(DroneID).motors.omega_max  LowerSaturationLimit=drone_params(DroneID).motors.omega_min
  prop_speed_scope : Scope
  wrench_scope : Scope  NumInputPorts=2
  p_world : Outport
  v_body : Outport  Port=2
  a_body : Outport  Port=3
  world2drone_quaternion : Outport  Port=4
  gyro : Outport  Port=5
  thrust : Outport  Port=6
  wires:
  calculate_wrench/1(thrust) -> wrench_scope/1, thrust/1, Translation/2(thrust)
  ESC/1(prop_acceleration) -> prop_speed/1
  desired_propellor_speeds/1 -> ESC/1(Omega_prop_d)
  prop_speed/1 -> prop_speed_scope/1, calculate_wrench/1(Omega_props), ESC/2(Omega_prop)
  calculate_wrench/2(moments) -> wrench_scope/2, Attitude/1(body moments)
  Attitude/1(attitude) -> world2drone_quaternion/1, Translation/1(attitude)
  Attitude/2(gyro) -> gyro/1
  Translation/3(body_v) -> v_body/1
  Translation/4(body_a) -> a_body/1
  Translation/1(p) -> p_world/1
  Translation/2(v) -> Scope/1

== system ErskineMultiDroneFormation/  Quadrotor13/Controller ==
  gyroscope : Inport
  attitude : Inport  Port=2
  velocity : Inport  Port=3
  position : Inport  Port=4
  input : Inport  Port=5
  Controller : MATLAB Function  TreatAsAtomicUnit=on
  Saturation : Saturate  UpperLimit=16  LowerLimit=3
  Saturation1 : Saturate  UpperLimit=0.1  LowerLimit=-0.1
  desired_prop_speed : MATLAB Function  TreatAsAtomicUnit=on
  prop_speeds : Outport
  wires:
  Controller/2(moments) -> Saturation1/1
  Saturation/1 -> desired_prop_speed/1(thrust)
  velocity/1 -> Controller/3(v)
  Saturation1/1 -> desired_prop_speed/2(moment)
  Controller/1(thrust) -> Saturation/1
  position/1 -> Controller/2(p)
  input/1 -> Controller/1(u)
  attitude/1 -> Controller/4(q)
  gyroscope/1 -> Controller/5(omega)
  desired_prop_speed/1(Omega_props) -> prop_speeds/1

== system ErskineMultiDroneFormation/  Quadrotor13/Quadrotor ==
  note: Quadrotor_dynamics
  note: Propeller Dynamics
  desired_propellor_speeds : Inport
  Attitude : Subsystem
  ESC : MATLAB Function  TreatAsAtomicUnit=on
  Scope : Scope
  Translation : Subsystem
  calculate_wrench : MATLAB Function  TreatAsAtomicUnit=on
  prop_speed : Integrator  InitialCondition=drone_params(DroneID).motors.omega0  LimitOutput=on  UpperSaturationLimit=drone_params(DroneID).motors.omega_max  LowerSaturationLimit=drone_params(DroneID).motors.omega_min
  prop_speed_scope : Scope
  wrench_scope : Scope  NumInputPorts=2
  p_world : Outport
  v_body : Outport  Port=2
  a_body : Outport  Port=3
  world2drone_quaternion : Outport  Port=4
  gyro : Outport  Port=5
  thrust : Outport  Port=6
  wires:
  calculate_wrench/1(thrust) -> wrench_scope/1, thrust/1, Translation/2(thrust)
  ESC/1(prop_acceleration) -> prop_speed/1
  desired_propellor_speeds/1 -> ESC/1(Omega_prop_d)
  prop_speed/1 -> prop_speed_scope/1, calculate_wrench/1(Omega_props), ESC/2(Omega_prop)
  calculate_wrench/2(moments) -> wrench_scope/2, Attitude/1(body moments)
  Attitude/1(attitude) -> world2drone_quaternion/1, Translation/1(attitude)
  Attitude/2(gyro) -> gyro/1
  Translation/3(body_v) -> v_body/1
  Translation/4(body_a) -> a_body/1
  Translation/1(p) -> p_world/1
  Translation/2(v) -> Scope/1

== system ErskineMultiDroneFormation/  Quadrotor2/Controller ==
  gyroscope : Inport
  attitude : Inport  Port=2
  velocity : Inport  Port=3
  position : Inport  Port=4
  input : Inport  Port=5
  Controller : MATLAB Function  TreatAsAtomicUnit=on
  Saturation : Saturate  UpperLimit=drone_params(DroneID).control.limits.thrust.max  LowerLimit=drone_params(DroneID).control.limits.thrust.min
  Saturation1 : Saturate  UpperLimit=0.1  LowerLimit=-0.1
  desired_prop_speed : MATLAB Function  TreatAsAtomicUnit=on
  prop_speeds : Outport
  wires:
  Controller/2(moments) -> Saturation1/1
  Saturation/1 -> desired_prop_speed/1(thrust)
  velocity/1 -> Controller/3(v)
  Saturation1/1 -> desired_prop_speed/2(moment)
  Controller/1(thrust) -> Saturation/1
  position/1 -> Controller/2(p)
  input/1 -> Controller/1(u)
  attitude/1 -> Controller/4(q)
  gyroscope/1 -> Controller/5(omega)
  desired_prop_speed/1(Omega_props) -> prop_speeds/1

== system ErskineMultiDroneFormation/  Quadrotor2/Quadrotor ==
  note: Quadrotor_dynamics
  note: Propeller Dynamics
  desired_propellor_speeds : Inport
  Attitude : Subsystem
  ESC : MATLAB Function  TreatAsAtomicUnit=on
  Scope : Scope
  Translation : Subsystem
  calculate_wrench : MATLAB Function  TreatAsAtomicUnit=on
  prop_speed : Integrator  InitialCondition=drone_params(DroneID).motors.omega0  LimitOutput=on  UpperSaturationLimit=drone_params(DroneID).motors.omega_max  LowerSaturationLimit=drone_params(DroneID).motors.omega_min
  prop_speed_scope : Scope
  wrench_scope : Scope  NumInputPorts=2
  p_world : Outport
  v_body : Outport  Port=2
  a_body : Outport  Port=3
  world2drone_quaternion : Outport  Port=4
  gyro : Outport  Port=5
  thrust : Outport  Port=6
  wires:
  calculate_wrench/1(thrust) -> wrench_scope/1, thrust/1, Translation/2(thrust)
  ESC/1(prop_acceleration) -> prop_speed/1
  desired_propellor_speeds/1 -> ESC/1(Omega_prop_d)
  prop_speed/1 -> prop_speed_scope/1, calculate_wrench/1(Omega_props), ESC/2(Omega_prop)
  calculate_wrench/2(moments) -> wrench_scope/2, Attitude/1(body moments)
  Attitude/1(attitude) -> world2drone_quaternion/1, Translation/1(attitude)
  Attitude/2(gyro) -> gyro/1
  Translation/3(body_v) -> v_body/1
  Translation/4(body_a) -> a_body/1
  Translation/1(p) -> p_world/1
  Translation/2(v) -> Scope/1

== system ErskineMultiDroneFormation/  Quadrotor3/Controller ==
  gyroscope : Inport
  attitude : Inport  Port=2
  velocity : Inport  Port=3
  position : Inport  Port=4
  input : Inport  Port=5
  Controller : MATLAB Function  TreatAsAtomicUnit=on
  Saturation : Saturate  UpperLimit=16  LowerLimit=3
  Saturation1 : Saturate  UpperLimit=0.1  LowerLimit=-0.1
  desired_prop_speed : MATLAB Function  TreatAsAtomicUnit=on
  prop_speeds : Outport
  wires:
  Controller/2(moments) -> Saturation1/1
  Saturation/1 -> desired_prop_speed/1(thrust)
  velocity/1 -> Controller/3(v)
  Saturation1/1 -> desired_prop_speed/2(moment)
  Controller/1(thrust) -> Saturation/1
  position/1 -> Controller/2(p)
  input/1 -> Controller/1(u)
  attitude/1 -> Controller/4(q)
  gyroscope/1 -> Controller/5(omega)
  desired_prop_speed/1(Omega_props) -> prop_speeds/1

== system ErskineMultiDroneFormation/  Quadrotor3/Quadrotor ==
  note: Quadrotor_dynamics
  note: Propeller Dynamics
  desired_propellor_speeds : Inport
  Attitude : Subsystem
  ESC : MATLAB Function  TreatAsAtomicUnit=on
  Scope : Scope
  Translation : Subsystem
  calculate_wrench : MATLAB Function  TreatAsAtomicUnit=on
  prop_speed : Integrator  InitialCondition=drone_params(DroneID).motors.omega0  LimitOutput=on  UpperSaturationLimit=drone_params(DroneID).motors.omega_max  LowerSaturationLimit=drone_params(DroneID).motors.omega_min
  prop_speed_scope : Scope
  wrench_scope : Scope  NumInputPorts=2
  p_world : Outport
  v_body : Outport  Port=2
  a_body : Outport  Port=3
  world2drone_quaternion : Outport  Port=4
  gyro : Outport  Port=5
  thrust : Outport  Port=6
  wires:
  calculate_wrench/1(thrust) -> wrench_scope/1, thrust/1, Translation/2(thrust)
  ESC/1(prop_acceleration) -> prop_speed/1
  desired_propellor_speeds/1 -> ESC/1(Omega_prop_d)
  prop_speed/1 -> prop_speed_scope/1, calculate_wrench/1(Omega_props), ESC/2(Omega_prop)
  calculate_wrench/2(moments) -> wrench_scope/2, Attitude/1(body moments)
  Attitude/1(attitude) -> world2drone_quaternion/1, Translation/1(attitude)
  Attitude/2(gyro) -> gyro/1
  Translation/3(body_v) -> v_body/1
  Translation/4(body_a) -> a_body/1
  Translation/1(p) -> p_world/1
  Translation/2(v) -> Scope/1

== system ErskineMultiDroneFormation/  Quadrotor4/Controller ==
  gyroscope : Inport
  attitude : Inport  Port=2
  velocity : Inport  Port=3
  position : Inport  Port=4
  input : Inport  Port=5
  Controller : MATLAB Function  TreatAsAtomicUnit=on
  Saturation : Saturate  UpperLimit=drone_params(DroneID).control.limits.thrust.max  LowerLimit=drone_params(DroneID).control.limits.thrust.min
  Saturation1 : Saturate  UpperLimit=0.1  LowerLimit=-0.1
  desired_prop_speed : MATLAB Function  TreatAsAtomicUnit=on
  prop_speeds : Outport
  wires:
  Controller/2(moments) -> Saturation1/1
  Saturation/1 -> desired_prop_speed/1(thrust)
  velocity/1 -> Controller/3(v)
  Saturation1/1 -> desired_prop_speed/2(moment)
  Controller/1(thrust) -> Saturation/1
  position/1 -> Controller/2(p)
  input/1 -> Controller/1(u)
  attitude/1 -> Controller/4(q)
  gyroscope/1 -> Controller/5(omega)
  desired_prop_speed/1(Omega_props) -> prop_speeds/1

== system ErskineMultiDroneFormation/  Quadrotor4/Quadrotor ==
  note: Quadrotor_dynamics
  note: Propeller Dynamics
  desired_propellor_speeds : Inport
  Attitude : Subsystem
  ESC : MATLAB Function  TreatAsAtomicUnit=on
  Scope : Scope
  Translation : Subsystem
  calculate_wrench : MATLAB Function  TreatAsAtomicUnit=on
  prop_speed : Integrator  InitialCondition=drone_params(DroneID).motors.omega0  LimitOutput=on  UpperSaturationLimit=drone_params(DroneID).motors.omega_max  LowerSaturationLimit=drone_params(DroneID).motors.omega_min
  prop_speed_scope : Scope
  wrench_scope : Scope  NumInputPorts=2
  p_world : Outport
  v_body : Outport  Port=2
  a_body : Outport  Port=3
  world2drone_quaternion : Outport  Port=4
  gyro : Outport  Port=5
  thrust : Outport  Port=6
  wires:
  calculate_wrench/1(thrust) -> wrench_scope/1, thrust/1, Translation/2(thrust)
  ESC/1(prop_acceleration) -> prop_speed/1
  desired_propellor_speeds/1 -> ESC/1(Omega_prop_d)
  prop_speed/1 -> prop_speed_scope/1, calculate_wrench/1(Omega_props), ESC/2(Omega_prop)
  calculate_wrench/2(moments) -> wrench_scope/2, Attitude/1(body moments)
  Attitude/1(attitude) -> world2drone_quaternion/1, Translation/1(attitude)
  Attitude/2(gyro) -> gyro/1
  Translation/3(body_v) -> v_body/1
  Translation/4(body_a) -> a_body/1
  Translation/1(p) -> p_world/1
  Translation/2(v) -> Scope/1

== system ErskineMultiDroneFormation/  Quadrotor5/Controller ==
  gyroscope : Inport
  attitude : Inport  Port=2
  velocity : Inport  Port=3
  position : Inport  Port=4
  input : Inport  Port=5
  Controller : MATLAB Function  TreatAsAtomicUnit=on
  Saturation : Saturate  UpperLimit=drone_params(DroneID).control.limits.thrust.max  LowerLimit=drone_params(DroneID).control.limits.thrust.min
  Saturation1 : Saturate  UpperLimit=0.1  LowerLimit=-0.1
  desired_prop_speed : MATLAB Function  TreatAsAtomicUnit=on
  prop_speeds : Outport
  wires:
  Controller/2(moments) -> Saturation1/1
  Saturation/1 -> desired_prop_speed/1(thrust)
  velocity/1 -> Controller/3(v)
  Saturation1/1 -> desired_prop_speed/2(moment)
  Controller/1(thrust) -> Saturation/1
  position/1 -> Controller/2(p)
  input/1 -> Controller/1(u)
  attitude/1 -> Controller/4(q)
  gyroscope/1 -> Controller/5(omega)
  desired_prop_speed/1(Omega_props) -> prop_speeds/1

== system ErskineMultiDroneFormation/  Quadrotor5/Quadrotor ==
  note: Quadrotor_dynamics
  note: Propeller Dynamics
  desired_propellor_speeds : Inport
  Attitude : Subsystem
  ESC : MATLAB Function  TreatAsAtomicUnit=on
  Scope : Scope
  Translation : Subsystem
  calculate_wrench : MATLAB Function  TreatAsAtomicUnit=on
  prop_speed : Integrator  InitialCondition=drone_params(DroneID).motors.omega0  LimitOutput=on  UpperSaturationLimit=drone_params(DroneID).motors.omega_max  LowerSaturationLimit=drone_params(DroneID).motors.omega_min
  prop_speed_scope : Scope
  wrench_scope : Scope  NumInputPorts=2
  p_world : Outport
  v_body : Outport  Port=2
  a_body : Outport  Port=3
  world2drone_quaternion : Outport  Port=4
  gyro : Outport  Port=5
  thrust : Outport  Port=6
  wires:
  calculate_wrench/1(thrust) -> wrench_scope/1, thrust/1, Translation/2(thrust)
  ESC/1(prop_acceleration) -> prop_speed/1
  desired_propellor_speeds/1 -> ESC/1(Omega_prop_d)
  prop_speed/1 -> prop_speed_scope/1, calculate_wrench/1(Omega_props), ESC/2(Omega_prop)
  calculate_wrench/2(moments) -> wrench_scope/2, Attitude/1(body moments)
  Attitude/1(attitude) -> world2drone_quaternion/1, Translation/1(attitude)
  Attitude/2(gyro) -> gyro/1
  Translation/3(body_v) -> v_body/1
  Translation/4(body_a) -> a_body/1
  Translation/1(p) -> p_world/1
  Translation/2(v) -> Scope/1

== system ErskineMultiDroneFormation/  Quadrotor6/Controller ==
  gyroscope : Inport
  attitude : Inport  Port=2
  velocity : Inport  Port=3
  position : Inport  Port=4
  input : Inport  Port=5
  Controller : MATLAB Function  TreatAsAtomicUnit=on
  Saturation : Saturate  UpperLimit=16  LowerLimit=3
  Saturation1 : Saturate  UpperLimit=0.1  LowerLimit=-0.1
  desired_prop_speed : MATLAB Function  TreatAsAtomicUnit=on
  prop_speeds : Outport
  wires:
  Controller/2(moments) -> Saturation1/1
  Saturation/1 -> desired_prop_speed/1(thrust)
  velocity/1 -> Controller/3(v)
  Saturation1/1 -> desired_prop_speed/2(moment)
  Controller/1(thrust) -> Saturation/1
  position/1 -> Controller/2(p)
  input/1 -> Controller/1(u)
  attitude/1 -> Controller/4(q)
  gyroscope/1 -> Controller/5(omega)
  desired_prop_speed/1(Omega_props) -> prop_speeds/1

== system ErskineMultiDroneFormation/  Quadrotor6/Quadrotor ==
  note: Quadrotor_dynamics
  note: Propeller Dynamics
  desired_propellor_speeds : Inport
  Attitude : Subsystem
  ESC : MATLAB Function  TreatAsAtomicUnit=on
  Scope : Scope
  Translation : Subsystem
  calculate_wrench : MATLAB Function  TreatAsAtomicUnit=on
  prop_speed : Integrator  InitialCondition=drone_params(DroneID).motors.omega0  LimitOutput=on  UpperSaturationLimit=drone_params(DroneID).motors.omega_max  LowerSaturationLimit=drone_params(DroneID).motors.omega_min
  prop_speed_scope : Scope
  wrench_scope : Scope  NumInputPorts=2
  p_world : Outport
  v_body : Outport  Port=2
  a_body : Outport  Port=3
  world2drone_quaternion : Outport  Port=4
  gyro : Outport  Port=5
  thrust : Outport  Port=6
  wires:
  calculate_wrench/1(thrust) -> wrench_scope/1, thrust/1, Translation/2(thrust)
  ESC/1(prop_acceleration) -> prop_speed/1
  desired_propellor_speeds/1 -> ESC/1(Omega_prop_d)
  prop_speed/1 -> prop_speed_scope/1, calculate_wrench/1(Omega_props), ESC/2(Omega_prop)
  calculate_wrench/2(moments) -> wrench_scope/2, Attitude/1(body moments)
  Attitude/1(attitude) -> world2drone_quaternion/1, Translation/1(attitude)
  Attitude/2(gyro) -> gyro/1
  Translation/3(body_v) -> v_body/1
  Translation/4(body_a) -> a_body/1
  Translation/1(p) -> p_world/1
  Translation/2(v) -> Scope/1

== system ErskineMultiDroneFormation/  Quadrotor7/Controller ==
  gyroscope : Inport
  attitude : Inport  Port=2
  velocity : Inport  Port=3
  position : Inport  Port=4
  input : Inport  Port=5
  Controller : MATLAB Function  TreatAsAtomicUnit=on
  Saturation : Saturate  UpperLimit=drone_params(DroneID).control.limits.thrust.max  LowerLimit=drone_params(DroneID).control.limits.thrust.min
  Saturation1 : Saturate  UpperLimit=0.1  LowerLimit=-0.1
  desired_prop_speed : MATLAB Function  TreatAsAtomicUnit=on
  prop_speeds : Outport
  wires:
  Controller/2(moments) -> Saturation1/1
  Saturation/1 -> desired_prop_speed/1(thrust)
  velocity/1 -> Controller/3(v)
  Saturation1/1 -> desired_prop_speed/2(moment)
  Controller/1(thrust) -> Saturation/1
  position/1 -> Controller/2(p)
  input/1 -> Controller/1(u)
  attitude/1 -> Controller/4(q)
  gyroscope/1 -> Controller/5(omega)
  desired_prop_speed/1(Omega_props) -> prop_speeds/1
